simulink model "psbbusbar"  (Simulink 6.0)
settings: Solver=ode15s  SolverMode=SingleTasking  StartTime=0.0  StopTime=10.0  RelTol=1e-3  AbsTol=1e-6
InitFcn:
  | powericon('psbinitsys',bdroot);
libraries: powerlib2 x10
settings Model: Creator=patrice  LastModifiedBy=batserve  ExtModeTrigMode=oneshot  ExtModeArmWhenConnect=off  ExtModeAutoUpdateStatusClock=off
settings DataIOCC: LimitDataPoints=off
settings OptimizationCC: BooleanDataType=off
settings DebuggingCC: SolverPrmCheckMsg=none
settings HardwareCC: TargetUnknown=on
settings RTWCC: TemplateMakefile=grt_unix.tmf

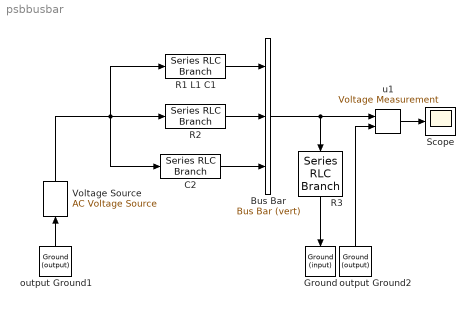
== system psbbusbar ==
  "Bus Bar " : powerlib2/Connectors/Bus Bar (vert)  Tag=PoWeRsYsTeMbLoCk  entrees=3  sorties=1  PSBOutputType=11111111111111111111111111111111111111111111111111111111111111111111111111111111111111111
  C2 : powerlib2/Elements/Series RLC Branch  Tag=PoWeRsYsTeMbLoCk  a=0  b=0  c=1  mesure=None  PSBOutputType=1
  Ground : powerlib2/Connectors/Ground (input)  Tag=PoWeRsYsTeMbLoCk  Orientation=down
  R1 L1 C1 : powerlib2/Elements/Series RLC Branch  Tag=PoWeRsYsTeMbLoCk  a=1  b=1e-03  c=1e-06  mesure=None  PSBOutputType=1
  R2 : powerlib2/Elements/Series RLC Branch  Tag=PoWeRsYsTeMbLoCk  a=1  b=0  c=inf  mesure=None  PSBOutputType=1
  R3 : powerlib2/Elements/Series RLC Branch  Tag=PoWeRsYsTeMbLoCk  Orientation=down  a=1  b=0  c=inf  mesure=None  PSBOutputType=1
  Scope : Scope
      settings: TickLabels=on  TimeRange=0.1  YMin=-50  YMax=50  DataFormat=Array
  Voltage Source : powerlib2/Electrical Sources/AC Voltage Source  Tag=PoWeRsYsTeMbLoCk  Description=source block  Orientation=up  A=50  P=0  F=60  stime=0  mesure=None  PSBOutputType=1
  output Ground1 : powerlib2/Connectors/Ground (output)  Tag=PoWeRsYsTeMbLoCk  Orientation=up  PSBOutputType=1
  output Ground2 : powerlib2/Connectors/Ground (output)  Tag=PoWeRsYsTeMbLoCk  Orientation=up  PSBOutputType=1
  u1 : powerlib2/Measurements/Voltage Measurement  Tag=PoWeRsYsTeMmEaSuReMeNt  PSBOutputType=0  PSBequivalent=1
  wires:
  R3/1 -> Ground/1
  "Bus Bar "/1 -> R3/1, u1/1
  output Ground2/1 -> u1/2
  u1/1 -> Scope/1
  output Ground1/1 -> Voltage Source/1
  R1 L1 C1/1 -> "Bus Bar "/1
  R2/1 -> "Bus Bar "/2
  C2/1 -> "Bus Bar "/3
  Voltage Source/1 -> R2/1, R1 L1 C1/1, C2/1
